simulink model "TestServoventil1"  (Simulink 9.3)
settings: Solver=VariableStepAuto  StartTime=0.0  StopTime=10.0  RelTol=1e-3
settings Model: Creator=wredi  LastModifiedBy=wredi
settings DataIOCC: SaveFormat=Dataset  SignalLoggingSaveFormat=Dataset  ReturnWorkspaceOutputs=on
settings OptimizationCC: LifeSpan=auto
settings DebuggingCC: UnderspecifiedInitializationDetection=Simplified  MergeDetectMultiDrivingBlocksExec=error  FcnCallInpInsideContextMsg=error  SFUnexpectedBacktrackingDiag=error  SFNoUnconditionalDefaultTransitionDiag=error  SFExecutionAtInitializationDiag=warning  ArithmeticOperatorsInVariantConditions=error
settings HardwareCC: ProdBitPerPointer=64  ProdBitPerSizeT=64  ProdBitPerPtrDiffT=64  ProdLargestAtomicFloat=Float  ProdIntDivRoundTo=Zero  ProdEndianess=LittleEndian  ProdWordSize=64  ProdHWDeviceType=Intel->x86-64 (Windows64)
settings ModelReferenceCC: PropagateSignalLabelsOutOfModel=on
settings SFSimCC: SimUseLocalCustomCode=on
settings RTWCC: RTWUseLocalCustomCode=on
settings CodeAppCC: StateflowObjectComments=off
settings GRTTargetCC: TargetLangStandard=C99 (ISO)  CombineOutputUpdateFcns=on  GRTInterface=off
settings ConfigComp: CovMetricSettings=dwe  CovHtmlReporting=off  CovSaveCumulativeToWorkspaceVar=off  CovSaveSingleToWorkspaceVar=off  CovExternalEMLEnable=on

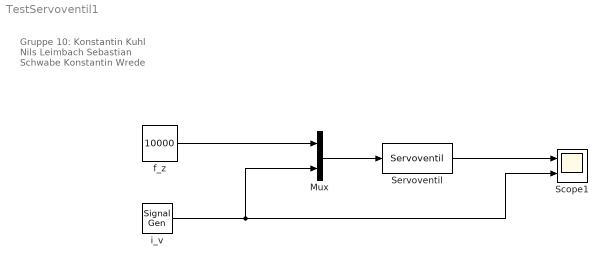
== system TestServoventil1 ==
  note: Gruppe 10:
      | Konstantin Kuhl
      | Nils Leimbach
      | Sebastian Schwabe
      | Konstantin Wrede
  Mux : Mux  Inputs=2
  Scope1 : Scope  NumInputPorts=2
  Servoventil : MATLABFcn  MATLABFcn=Servoventil  OutputDimensions=1
  f_z : Constant  Value=10000
  i_v : SignalGenerator  WaveForm=square  Amplitude=5  Units=rad/sec
  wires:
  Mux/1 -> Servoventil/1
  f_z/1 -> Mux/1
  Servoventil/1 -> Scope1/1
  i_v/1 -> Scope1/2, Mux/2
